simulink library "PlateShield"  (R2025b)
settings: Solver=VariableStepAuto  StartTime=0.0  StopTime=10.0  RelTol=1e-3
libraries: arduinolib x3, $bdroot x3
settings Model: Creator=irach  LastModifiedBy=irach

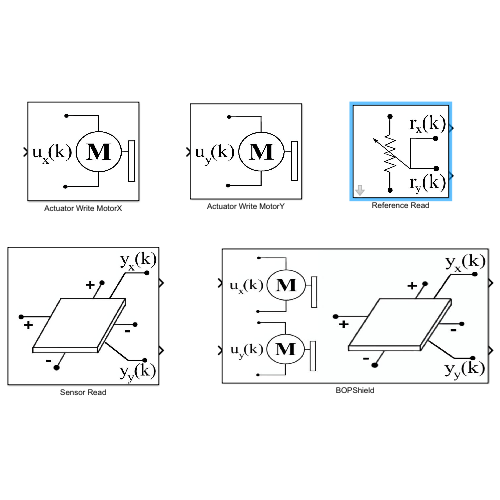
[thumbnail: Simulink's stored preview of the top-level diagram]
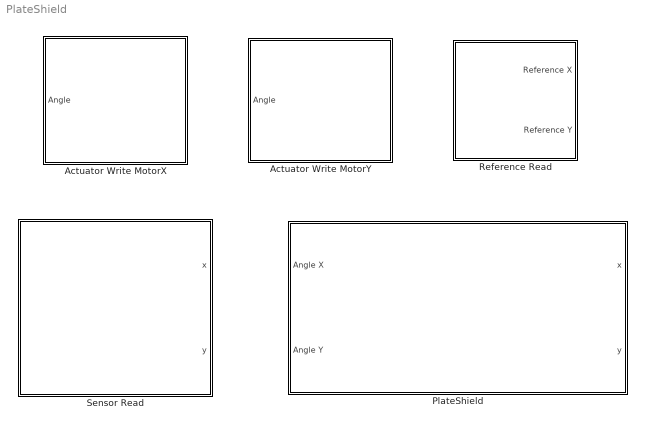
== system PlateShield ==
  Actuator Write MotorX : Subsystem
      mask Display: image('motorx.jpg');
  Actuator Write MotorY : Subsystem
      mask Display: image('motory.jpg');
  PlateShield : Subsystem
      mask Display: image('bop.jpg');
  Reference Read : Subsystem  mask{mode=Center}
      mask prompts: mode "Regime"
      mask TypeOptions mode: Center | Circle | Oval
      mask Display: image('reference.jpg');
  Sensor Read : Subsystem
      mask Display: image('sensor.jpg');

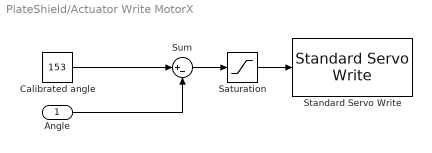
== system PlateShield/Actuator Write MotorX ==
  Angle : Inport
  Calibrated angle : Constant  Value=153
  Saturation : Saturate  UpperLimit=180  LowerLimit=0
  Standard Servo Write : arduinolib/Standard Servo Write  pinNumber=9  ServoIndex=0  blockPlatform=ARDUINO
  Sum : Sum  Inputs=|+-
  wires:
  Sum/1 -> Saturation/1
  Calibrated angle/1 -> Sum/1
  Angle/1 -> Sum/2
  Saturation/1 -> Standard Servo Write/1

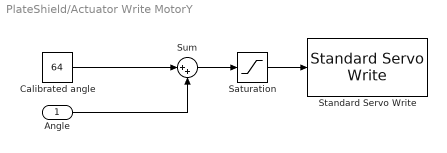
== system PlateShield/Actuator Write MotorY ==
  Angle : Inport
  Calibrated angle : Constant  Value=64
  Saturation : Saturate  UpperLimit=180  LowerLimit=0
  Standard Servo Write : arduinolib/Standard Servo Write  pinNumber=8  ServoIndex=0  blockPlatform=ARDUINO
  Sum : Sum  Inputs=|++
  wires:
  Calibrated angle/1 -> Sum/1
  Angle/1 -> Sum/2
  Sum/1 -> Saturation/1
  Saturation/1 -> Standard Servo Write/1

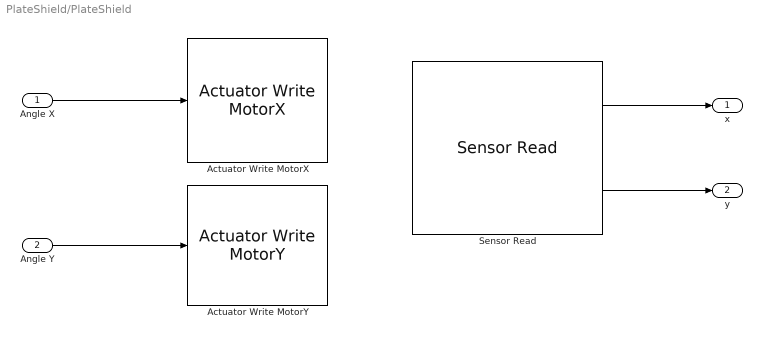
== system PlateShield/PlateShield ==
  Angle X : Inport
  Angle Y : Inport  Port=2
  Actuator Write MotorX : $bdroot/Actuator Write MotorX  SystemSampleTime=-1  VariantActivationTime=update diagram  EmptyChoice=off  PassThrough=off  PassThroughVariantControl=(default)  EmptyChoiceVariantControl=(default)  AllowFlexibleInterface=on  Latency=0  AutoFrameSizeCalculation=off
  Actuator Write MotorY : $bdroot/Actuator Write MotorY  SystemSampleTime=-1  VariantActivationTime=update diagram  EmptyChoice=off  PassThrough=off  PassThroughVariantControl=(default)  EmptyChoiceVariantControl=(default)  AllowFlexibleInterface=on  Latency=0  AutoFrameSizeCalculation=off
  Sensor Read : $bdroot/Sensor Read  SystemSampleTime=-1  VariantActivationTime=update diagram  EmptyChoice=off  PassThrough=off  PassThroughVariantControl=(default)  EmptyChoiceVariantControl=(default)  AllowFlexibleInterface=on  Latency=0  AutoFrameSizeCalculation=off
  x : Outport
  y : Outport  Port=2
  wires:
  Angle Y/1 -> Actuator Write MotorY/1
  Angle X/1 -> Actuator Write MotorX/1
  Sensor Read/1 -> x/1
  Sensor Read/2 -> y/1

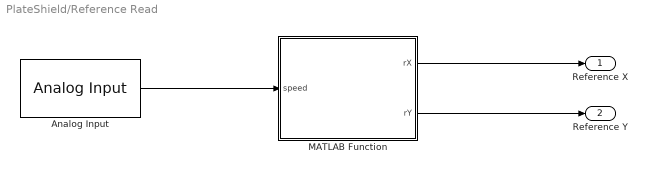
== system PlateShield/Reference Read ==
  Analog Input : arduinolib/Analog Input  pinNumber=4  ReadResultsOnly=off  ConversionTriggerSource=Software  ExternalTriggerType=uint32( 0 )  OutputDataType=uint16  EnableConversionCompleteNotify=off  EnableOuputStatus=off  SampleTime=0.05  blockPlatform=arduino
  MATLAB Function : MATLAB Function  TreatAsAtomicUnit=on
  Reference X : Outport
  Reference Y : Outport  Port=2
  wires:
  MATLAB Function/1(rX) -> Reference X/1
  MATLAB Function/2(rY) -> Reference Y/1
  Analog Input/1 -> MATLAB Function/1(speed)

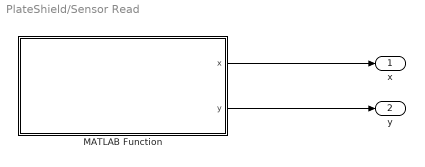
== system PlateShield/Sensor Read ==
  MATLAB Function : MATLAB Function  TreatAsAtomicUnit=on
  x : Outport
  y : Outport  Port=2
  wires:
  MATLAB Function/2(y) -> y/1
  MATLAB Function/1(x) -> x/1

== matlab function PlateShield/Reference Read/MATLAB Function ==
  data: rX output; speed input; rY output; mode parameter uint8 size=1
function [rX, rY] = fcn(speed, mode)
persistent i lastTime rXprev rYprev simTime oldMode

if isempty(i)
    i = uint8(1);
    lastTime = uint32(0);
    rXprev = single(51);
    rYprev = single(30);
    simTime = uint32(0);
    oldMode = uint8(0);
end

CircleX = single([76 75 74 71 68 64 59 54 49 44 39 34 30 27 25 26 26 27 30 34 39 44 49 54 59 64 68 71 74 75 76 76]);
CircleY = single([30 35 40 45 49 53 55 56 56 55 53 49 45 40 35 30 25 20 15 11 7 5 4 4 5 7 11 15 20 25 30 30]);

OvalX = single([76 76 75 74 69 66 61 56 51 46 41 36 33 30 27 26 26 26 27 30 33 36 41 46 51 56 61 66 69 74 75 76]);
OvalY = single([30 33 36 38 41 43 44 45 45 45 44 43 41 38 36 33 30 27 24 22 19 17 16 15 15 15 16 17 19 22 24 27]);

choice = uint8(mode);

speedValue = single(speed);
speedValue = min(max(speedValue, single(0)), single(1023));

timeInterval = uint32(50 + speedValue * single(50) / single(1023));

nowTime = uint32(0);

if coder.target('Rtw')
    coder.cinclude('Arduino.h');
    nowTime = coder.ceval('millis');
else
    simTime = simTime + uint32(50);
    nowTime = simTime;
end
if choice ~= oldMode
    i = uint8(1);
    lastTime = nowTime;
    rXprev = single(51);
    rYprev = single(30);
    oldMode = choice;
end

if choice == 1

    rX = single(51);
    rY = single(30);

elseif choice == 2

    if nowTime - lastTime >= timeInterval
        rXprev = CircleX(i);
        rYprev = CircleY(i);

        i = i + uint8(1);
        if i > 32
            i = uint8(1);
        end

        lastTime = nowTime;
    end

    rX = rXprev;
    rY = rYprev;

elseif choice == 3

    if nowTime - lastTime >= timeInterval
        rXprev = OvalX(i);
        rYprev = OvalY(i);

        i = i + uint8(1);
        if i > 32
            i = uint8(1);
        end

        lastTime = nowTime;
    end

    rX = rXprev;
    rY = rYprev;

else

    rX = single(51);
    rY = single(30);

end

== matlab function PlateShield/Sensor Read/MATLAB Function ==
  data: x output; y output
function [x, y] = sensorRead()

% Arduino Mega analog pins:
% A0 = 54, A1 = 55, A2 = 56, A3 = 57
X1 = uint8(54);  % A0
Y1 = uint8(55);  % A1
X2 = uint8(56);  % A2
Y2 = uint8(57);  % A3

Xmin = single(89);
Xmax = single(948);
Ymin = single(137);
Ymax = single(842);

Xraw = uint16(0);
Yraw = uint16(0);

if coder.target('Rtw')

    coder.cinclude('Arduino.h');

   
    coder.ceval('pinMode', X1, uint8(1));
    coder.ceval('pinMode', X2, uint8(1)); 
    coder.ceval('pinMode', Y1, uint8(0)); 
    coder.ceval('pinMode', Y2, uint8(0)); 

    coder.ceval('digitalWrite', X1, uint8(1)); 
    coder.ceval('digitalWrite', X2, uint8(0)); 

    coder.ceval('delayMicroseconds', uint16(50));

    Xraw = coder.ceval('analogRead', Y1);

   
    coder.ceval('pinMode', Y1, uint8(1)); 
    coder.ceval('pinMode', Y2, uint8(1));
    coder.ceval('pinMode', X1, uint8(0)); 
    coder.ceval('pinMode', X2, uint8(0)); 

    coder.ceval('digitalWrite', Y1, uint8(1)); 
    coder.ceval('digitalWrite', Y2, uint8(0)); 

    coder.ceval('delayMicroseconds', uint16(50));

    Yraw = coder.ceval('analogRead', X1);

else

    Xraw = uint16(512);
    Yraw = uint16(512);

end

x = single((single(Xraw) - Xmin) * single(103) / (Xmax - Xmin));
y = single((single(Yraw) - Ymin) * single(60) / (Ymax - Ymin));

x = min(max(x, single(0)), single(103));
y = min(max(y, single(0)), single(60));
